simulink model "nav_final4"  (R2024b)
settings: Solver=ode1  StartTime=0.0  StopTime=inf  FixedStep=Controller_Sample_Time  RelTol=1e-3  EnableMultiTasking=on
StartFcn:
  | cmd = 'powershell -command "$p = Start-Process python ''C:\Users\desqu\Downloads\servidor_yolo.py'' -PassThru; $p.Id"';
  | [~, pid] = system(cmd);
  | 
  | pid = str2double(strtrim(pid));
  | assignin('base','python_pid',pid);
StopFcn:
  | pid = evalin('base','python_pid');
  | system(['taskkill /PID ' num2str(pid) ' /F']);
undefined symbols (not defined in the file): AAAF5050, angles_qcar2, cal_pos, Controller_Sample_Time, CSI_Sample_Time, goalNode, GyroKF_P0, GyroKF_Q, GyroKF_R, GyroKF_X0, HIL, ImageDisplay_Sample_Time, Initialization_Time, K12, LiDAR_Sample_Time, MC, nodes, path_x4, path_x_dijkstra, path_x_smooth, path_y_dijkstra, path_y_smooth, Point, qc_get_step_size, qcar2_lidar_to_body_rotation, qcar2_lidar_to_map_rotation, qcar2_virtual_to_physical_lidar_rotation, QCarEKF_L, QCarEKF_P0, QCarEKF_Q, QCarEKF_R_combined, QCarEKF_R_heading, QcarKF_X0, range_qcar2, RealSense_Sample_Time, segmentos_der, segmentos_izq, steering_Kd, steering_Kp
libraries: quarc_library x36, simulink x3, simulink_extras x3
(part 3 of 3)

== matlab function nav_final4/trafficSignalLogic/trafficSignalLogic ==
  settings: updateMethod=DISCRETE
  data: speed_in input; speed_out output; detections input; t input; stop_ligth output; pedestrian_flag input; traffic_light_flag input; finished_flag input
function [speed_out, stop_ligth]= trafficSignsLogic(speed_in, detections, t, pedestrian_flag, traffic_light_flag, finished_flag)

persistent stop_active t_start stop_done
persistent yield_active t_yield_start yield_done
persistent person_active t_person_start person_phase person_done


if isempty(stop_active)
    stop_active = false;
    t_start = 0;
    stop_done = false;

    yield_active = false;
    t_yield_start = 0;
    yield_done = false;

    % person
    person_active = false;
    t_person_start = 0;
    person_phase = 0;
    person_done = false;
end


speed_out = speed_in;

stop_detected = false;
yield_detected = false;
round_detected = false;
person_detected = false;
stop_ligth = 0;

for i = 1:10

    class_id = detections(1,i);
    prob     = detections(2,i);
    dist     = detections(7,i);

    x1 = detections(3,i);
    x2 = detections(5,i);
    cx = (x1 + x2)/2;

    frontal = abs(cx - 320) < 100;
    right_side = cx > 360;

    % STOP
    if class_id == 5 && prob > 0.9 && dist < 1.3 && frontal
        stop_detected = true;
    end

    % YIELD
    if class_id == 7 && prob > 0.9 && dist < 1.5 && frontal
        yield_detected = true;
    end

    % ROUND
    if class_id == 4 && prob > 0.8 && dist < 2.0 && frontal
        round_detected = true;
    end

    % PERSON (right side)
    if class_id == 2 && prob > 0.8 && dist < 7.3 && right_side
        person_detected = true;
    end

end


% PEDESTRIAN STOP (HIGH PRIORITY)
if pedestrian_flag == 1
    speed_out = 0;
    stop_ligth = 1;
    return;
end

if finished_flag == 1
    speed_out = 0;
    stop_ligth = 1;
    return;
end

if traffic_light_flag == 1
    speed_out = 0;
    stop_ligth = 1;
    return;
end

% STOP
if stop_detected && ~stop_active && ~stop_done
    stop_active = true;
    stop_ligth = 1;
    t_start = t;
end

if stop_active
    if (t - t_start) < 5
        speed_out = 0;
        return;
    else
        stop_ligth = 0;
        stop_active = false;
        stop_done = true;
    end
end

if ~stop_detected
    stop_done = false;
end

% YIELD
if yield_detected && ~yield_active && ~yield_done
    yield_active = true;
    t_yield_start = t;
end

if yield_active
    if (t - t_yield_start) < 2
        speed_out = 0;
        stop_ligth = 1;
        return;
    else
        yield_active = false;
        stop_ligth = 0;
        yield_done = true;
    end
end

if ~yield_detected
    yield_done = false;
end

% PERSON (pickup)
if person_detected && ~person_active && ~person_done
    person_active = true;
    t_person_start = t;
    person_phase = 1;
end

if person_active

    dt = t - t_person_start;

    % Phase 1: move forward
    if dt < 3
        speed_out = speed_in; 

    % Phase 2: stop
    elseif dt < 6
        speed_out = 0;
        stop_ligth = 1;
    else
        person_active = false;
        person_done = true;
        stop_ligth = 0;
    end

    return;
end

% ROUND
if round_detected
    speed_out = 0.5 * speed_in;
end

end

== matlab function nav_final4/Collision Avoidance System (CAS)/avoidObstacle ==
  settings: updateMethod=DISCRETE
  data: steering_in input; steering_out output; detections input; t input; direction output
function [steering_out, direction]= avoidCone(steering_in, detections, t)

    persistent avoid_active t_start

    if isempty(avoid_active)
        avoid_active = false;
        t_start = 0;
    end

    % Parámetros de la maniobra (ajustar según pruebas)
    T_total = 3.0; % Duración total de la maniobra en segundos
    Amp = 0.4;     % Amplitud máxima del giro para esquivar  0.4

    cone_detected = false;
    direction = 0;

    %  lógica de detección actual (simplificada para el ejemplo)
    for i = 1:size(detections, 2)
        class_id = detections(1,i);
        prob     = detections(2,i);
        dist     = detections(7,i);
        
        % Si detectamos cono a menos de n metros
        if class_id == 0 && prob > 0.85 && dist < 2.0 
            cone_detected = true;
            
            break;
        end
    end

    % Disparar la maniobra
    %if cone_detected && ~avoid_active
    if cone_detected && ~avoid_active 
        avoid_active = true;
        
        t_start = t;
    end

    if avoid_active
        dt = t - t_start;
        
        
        if dt < T_total
            direction = 1;
            % Generamos una onda senoidal completa para entrar y salir
            % Esto crea un movimiento de "S" suave: izquierda -> derecha -> centro
            steering_avoid = Amp * sin(2 * pi * dt / T_total);
            
            % Prioridad: Ignoramos el steering_in del path original 
            % para evitar que el saturador nos bloquee la maniobra.
            steering_out = steering_avoid; 
        else
            avoid_active = false;
     
            direction = 0;
            steering_out = steering_in;
        end
    else
        steering_out = steering_in;
        direction = 0;
    end
end
